simulink model "LPL_Hopper_Model"  (R2024b)
settings: Solver=VariableStepAuto  StartTime=0.0  StopTime=10.0  RelTol=1e-3
values from neighbouring files (symbols this model uses):
  S_Eb = [(-3/4)*He*me; 0; 0]    [HopperSimDriverScript.m]
  S_TD = [x_cg*mf; 0 ; 0]    [HopperSimDriverScript.m]
  THETA_IC = [0 0 0]    [HopperSimDriverScript.m]
  v_b_0 = [1 0 0]'    [HopperSimDriverScript.m]
libraries: matrix_library x5, sharedtransform x2, aerolibutil x1, sharedutil x1
settings Model: Creator=enson  LastModifiedBy=enson
settings RTWCC: GPUComputeCapability=3.5

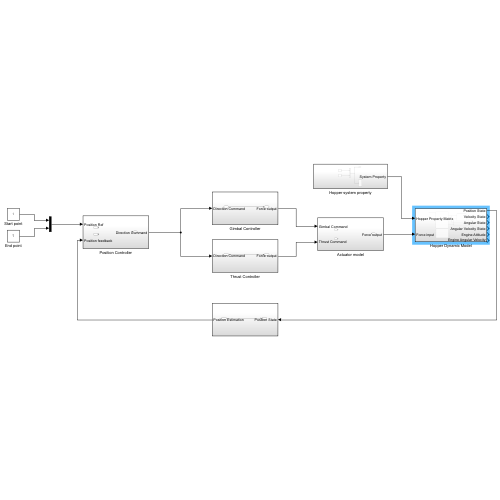
[thumbnail: Simulink's stored preview of the top-level diagram]
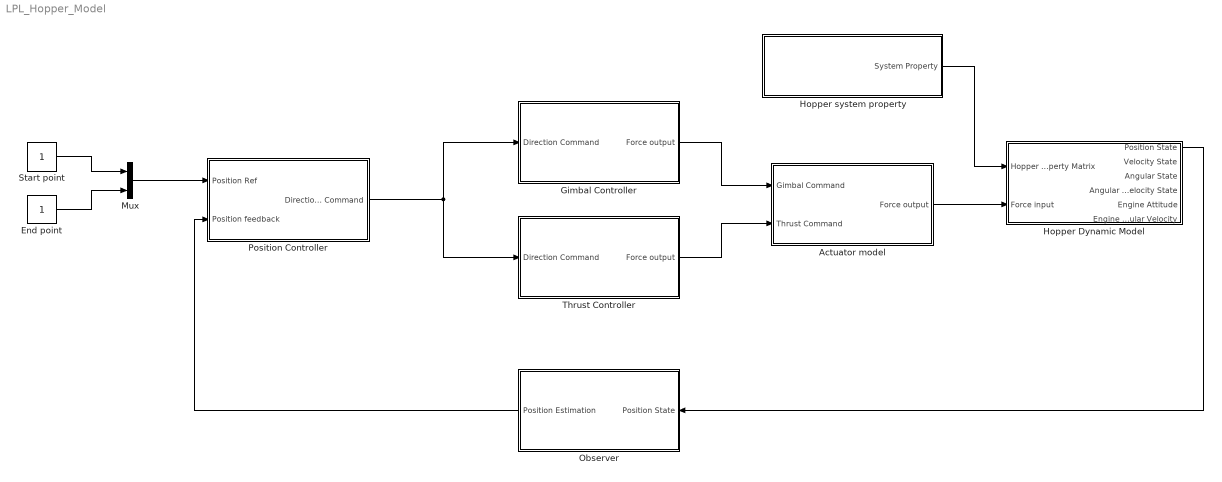
== system LPL_Hopper_Model ==
  Actuator model : Subsystem
  End point : Constant
  Gimbal Controller : Subsystem
  Hopper Dynamic Model : Subsystem
  Hopper system property : Subsystem
  Mux : Mux  Inputs=2
  Observer : Subsystem
  Position Controller : Subsystem
  Start point : Constant
  Thrust Controller : Subsystem
  wires:
  Mux/1 -> Position Controller/1(Position Ref)
  Start point/1 -> Mux/1
  End point/1 -> Mux/2
  Hopper Dynamic Model/1(Position State) -> Observer/1(Position State)
  Observer/1(Position Estimation) -> Position Controller/2(Position feedback)
  Position Controller/1(Direction Command) -> Gimbal Controller/1(Direction Command), Thrust Controller/1(Direction Command)
  Gimbal Controller/1(Force output) -> Actuator model/1(Gimbal Command)
  Thrust Controller/1(Force output) -> Actuator model/2(Thrust Command)
  Actuator model/1(Force output) -> Hopper Dynamic Model/2(Force input)
  Hopper system property/1(System Property) -> Hopper Dynamic Model/1(Hopper Property Matrix)

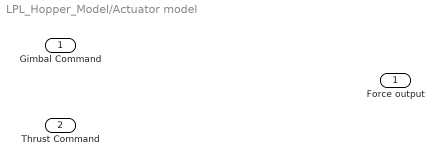
== system LPL_Hopper_Model/Actuator model ==
  Gimbal Command : Inport
  Thrust Command : Inport  Port=2
  Force output : Outport

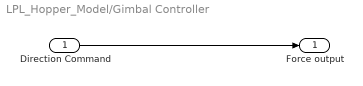
== system LPL_Hopper_Model/Gimbal Controller ==
  Direction Command : Inport
  Force output : Outport
  wires:
  Direction Command/1 -> Force output/1

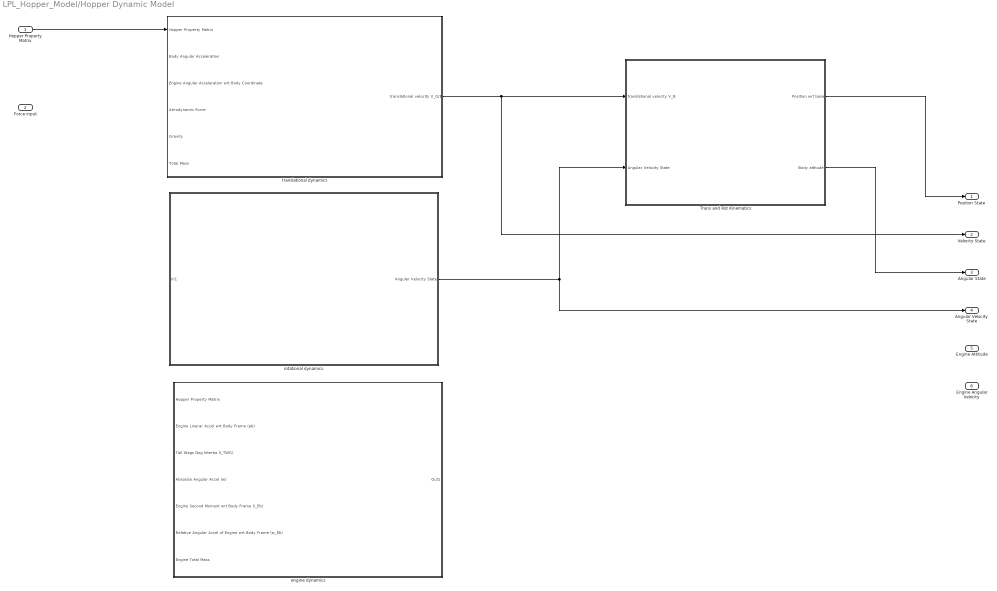
== system LPL_Hopper_Model/Hopper Dynamic Model ==
  Hopper Property Matrix : Inport
  Force input : Inport  Port=2
  Trans and Rot Kinematics : Subsystem
  engine dynamics : Subsystem
  rotational dynamics : Subsystem
  translational dynamics : Subsystem
  Position State : Outport
  Velocity State : Outport  Port=2
  Angular State : Outport  Port=3
  Angular Velocity State : Outport  Port=4
  Engine Attitude : Outport  Port=5
  Engine Angular Velocity : Outport  Port=6
  wires:
  Hopper Property Matrix/1 -> translational dynamics/1(Hopper Property Matrix)
  rotational dynamics/1(Angular Velocity State) -> Angular Velocity State/1, Trans and Rot Kinematics/2(Angular Velocity State)
  translational dynamics/1(translational velocity V_O/E) -> Velocity State/1, Trans and Rot Kinematics/1(translational velocity V_B)
  Trans and Rot Kinematics/1(Position wrt base) -> Position State/1
  Trans and Rot Kinematics/2(Body attitude) -> Angular State/1

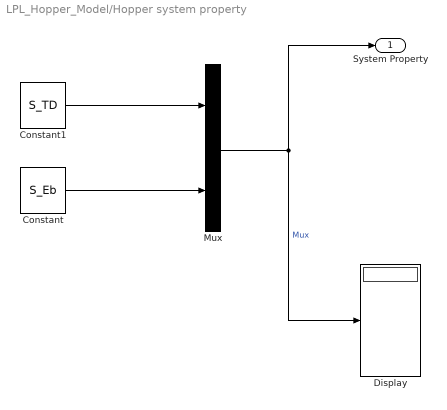
== system LPL_Hopper_Model/Hopper system property ==
  Constant : Constant  Value=S_Eb  VectorParams1D=off
  Constant1 : Constant  Value=S_TD  VectorParams1D=off
  Display : Display
  Mux : Mux  Inputs=2
  System Property : Outport
  wires:
  Mux/1 -> Display/1, System Property/1  "Mux"
  Constant/1 -> Mux/2
  Constant1/1 -> Mux/1

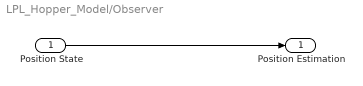
== system LPL_Hopper_Model/Observer ==
  Position State : Inport
  Position Estimation : Outport
  wires:
  Position State/1 -> Position Estimation/1

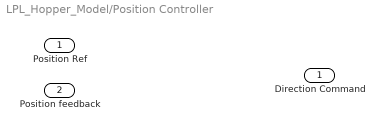
== system LPL_Hopper_Model/Position Controller ==
  Position Ref : Inport
  Position feedback : Inport  Port=2
  Direction Command : Outport

== system LPL_Hopper_Model/Thrust Controller ==
  Direction Command : Inport
  Force output : Outport
  wires:
  Direction Command/1 -> Force output/1

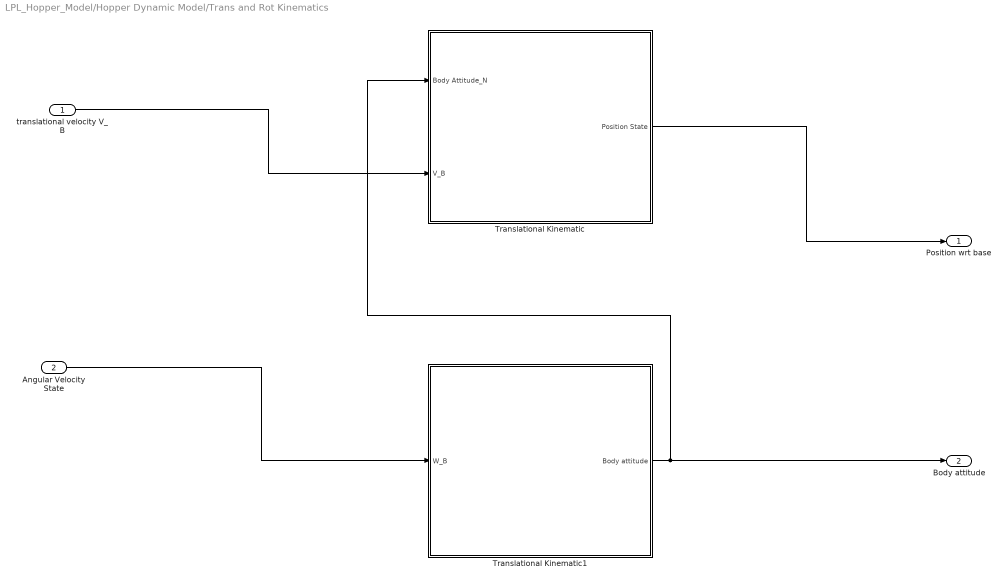
== system LPL_Hopper_Model/Hopper Dynamic Model/Trans and Rot Kinematics ==
  translational velocity V_B : Inport
  Angular Velocity State : Inport  Port=2
  Translational Kinematic : Subsystem
  Translational Kinematic1 : Subsystem
  Position wrt base : Outport
  Body attitude : Outport  Port=2
  wires:
  translational velocity V_B/1 -> Translational Kinematic/2(V_B)
  Translational Kinematic1/1(Body attitude) -> Body attitude/1, Translational Kinematic/1(Body Attitude_N)
  Angular Velocity State/1 -> Translational Kinematic1/1(W_B)
  Translational Kinematic/1(Position State) -> Position wrt base/1

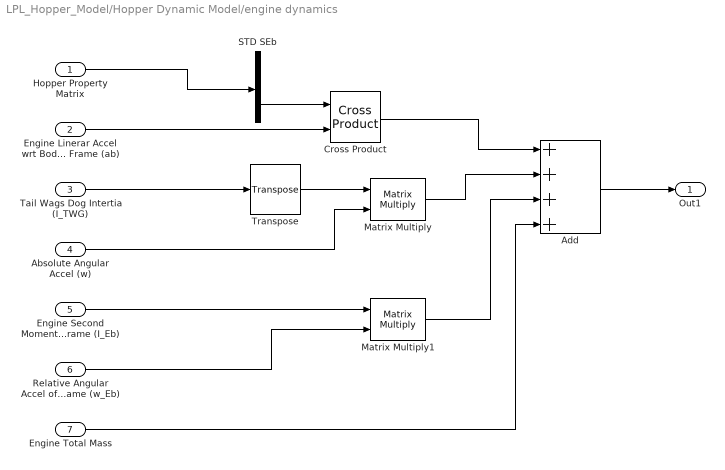
== system LPL_Hopper_Model/Hopper Dynamic Model/engine dynamics ==
  Hopper Property Matrix : Inport
  Engine Linerar Accel wrt Body Frame (ab) : Inport  Port=2
  Tail Wags Dog Intertia (I_TWG) : Inport  Port=3
  Absolute Angular Accel (w) : Inport  Port=4
  Engine Second Moment wrt Body Frame (I_Eb) : Inport  Port=5
  Relative Angular Accel of Engine wrt Body Frame (w_Eb) : Inport  Port=6
  Engine Total Mass : Inport  Port=7
  Add : Sum  Inputs=++++
  Cross Product : matrix_library/Cross Product
  Matrix Multiply : Product  Multiplication=Matrix(*)
  Matrix Multiply1 : Product  Multiplication=Matrix(*)
  STD SEb : Demux  Outputs=2
  Transpose : matrix_library/Transpose
  Out1 : Outport
  wires:
  Hopper Property Matrix/1 -> STD SEb/1
  STD SEb/2 -> Cross Product/1
  Engine Linerar Accel wrt Body Frame (ab)/1 -> Cross Product/2
  Cross Product/1 -> Add/1
  Tail Wags Dog Intertia (I_TWG)/1 -> Transpose/1
  Add/1 -> Out1/1
  Transpose/1 -> Matrix Multiply/1
  Absolute Angular Accel (w)/1 -> Matrix Multiply/2
  Matrix Multiply/1 -> Add/2
  Engine Second Moment wrt Body Frame (I_Eb)/1 -> Matrix Multiply1/1
  Relative Angular Accel of Engine wrt Body Frame (w_Eb)/1 -> Matrix Multiply1/2
  Matrix Multiply1/1 -> Add/3
  Engine Total Mass/1 -> Add/4

== system LPL_Hopper_Model/Hopper Dynamic Model/rotational dynamics ==
  In1 : Inport
  Angular Velocity State : Outport
  wires:
  In1/1 -> Angular Velocity State/1

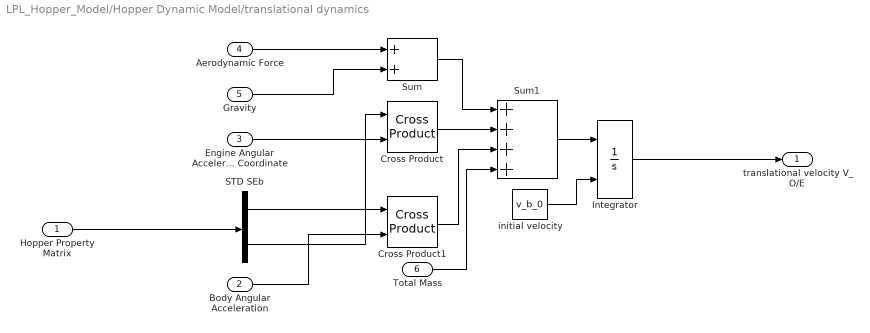
== system LPL_Hopper_Model/Hopper Dynamic Model/translational dynamics ==
  Hopper Property Matrix : Inport
  Body Angular Acceleration : Inport  Port=2
  Engine Angular Acceleration wrt Body Coordinate : Inport  Port=3
  Aerodynamic Force : Inport  Port=4
  Gravity : Inport  Port=5
  Total Mass : Inport  Port=6
  Cross Product : matrix_library/Cross Product
  Cross Product1 : matrix_library/Cross Product
  Integrator : Integrator  InitialConditionSource=external
  STD SEb : Demux  Outputs=2
  Sum : Sum
  Sum1 : Sum  Inputs=++++
  initial velocity : Constant  Value=v_b_0
  translational velocity V_O/E : Outport
  wires:
  Hopper Property Matrix/1 -> STD SEb/1
  Gravity/1 -> Sum/2
  Engine Angular Acceleration wrt Body Coordinate/1 -> Cross Product/2
  Aerodynamic Force/1 -> Sum/1
  STD SEb/2 -> Cross Product/1
  STD SEb/1 -> Cross Product1/1
  Body Angular Acceleration/1 -> Cross Product1/2
  Sum/1 -> Sum1/1
  Total Mass/1 -> Sum1/4
  Cross Product/1 -> Sum1/2
  Cross Product1/1 -> Sum1/3
  Sum1/1 -> Integrator/1
  initial velocity/1 -> Integrator/2
  Integrator/1 -> translational velocity V_O/E/1

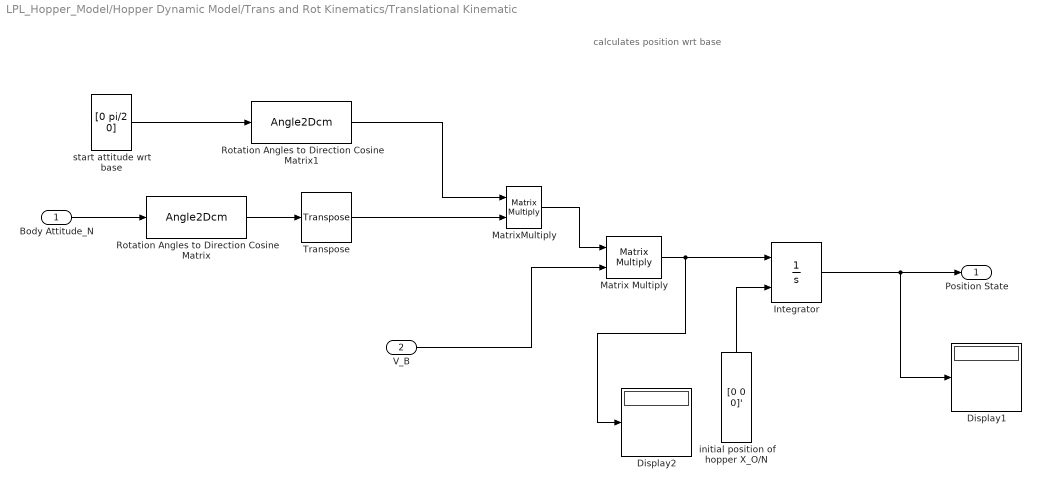
== system LPL_Hopper_Model/Hopper Dynamic Model/Trans and Rot Kinematics/Translational Kinematic ==
  note: calculates position wrt base
  Body Attitude_N : Inport
  V_B : Inport  Port=2
  Display1 : Display
  Display2 : Display
  Integrator : Integrator  InitialConditionSource=external
  Matrix Multiply : Product  Multiplication=Matrix(*)
  MatrixMultiply : Product  Multiplication=Matrix(*)
  Rotation Angles to Direction Cosine Matrix : Angle2Dcm
      settings: AttributesFormatString=Rotation Order: %<rotationOrder>
  Rotation Angles to Direction Cosine Matrix1 : Angle2Dcm
      settings: AttributesFormatString=Rotation Order: %<rotationOrder>
  Transpose : matrix_library/Transpose
  initial position of hopper X_O/N : Constant  Value=[0 0 0]'
  start attitude wrt base : Constant  Value=[0 pi/2 0]
  Position State : Outport
  wires:
  Matrix Multiply/1 -> Display2/1, Integrator/1
  initial position of hopper X_O/N/1 -> Integrator/2
  Integrator/1 -> Display1/1, Position State/1
  V_B/1 -> Matrix Multiply/2
  Body Attitude_N/1 -> Rotation Angles to Direction Cosine Matrix/1
  Rotation Angles to Direction Cosine Matrix/1 -> Transpose/1
  start attitude wrt base/1 -> Rotation Angles to Direction Cosine Matrix1/1
  Rotation Angles to Direction Cosine Matrix1/1 -> MatrixMultiply/1
  Transpose/1 -> MatrixMultiply/2
  MatrixMultiply/1 -> Matrix Multiply/1

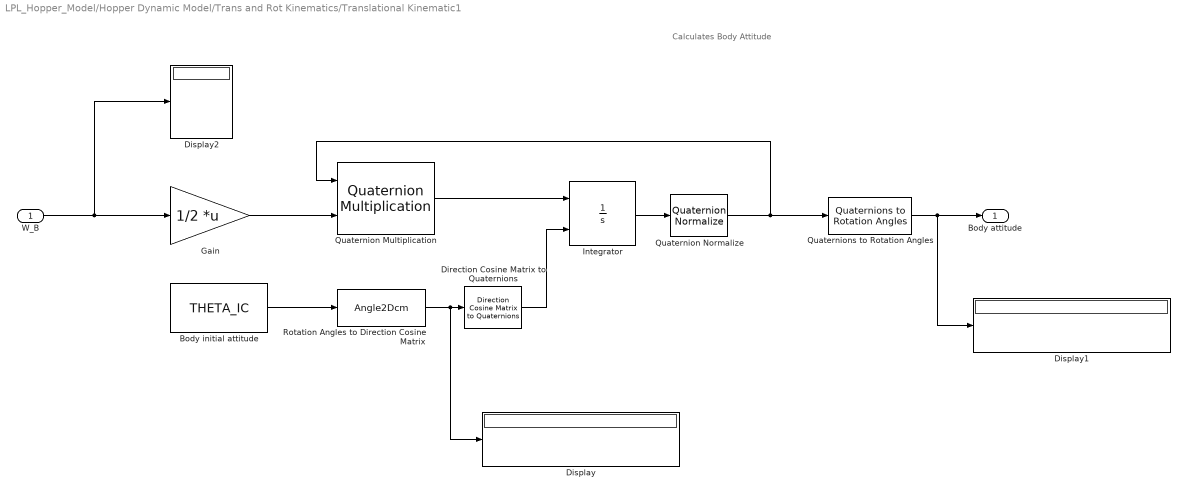
== system LPL_Hopper_Model/Hopper Dynamic Model/Trans and Rot Kinematics/Translational Kinematic1 ==
  note: Calculates Body Attitude
  W_B : Inport
  Body initial attitude : Constant  Value=THETA_IC  VectorParams1D=off
  Direction Cosine Matrix to Quaternions : sharedtransform/Direction Cosine Matrix  to Quaternions  aMode=0  action=None  tolerance=eps(2)
  Display : Display
  Display1 : Display
  Display2 : Display
  Gain : Gain  Gain=1/2  Multiplication=Matrix(K*u)
  Integrator : Integrator  InitialConditionSource=external
  Quaternion Multiplication : aerolibutil/Quaternion Multiplication
  Quaternion Normalize : sharedutil/Quaternion Normalize  aMode=aMode
  Quaternions to Rotation Angles : sharedtransform/Quaternions to Rotation Angles  rotationOrder=ZYX  aMode=aMode
  Rotation Angles to Direction Cosine Matrix : Angle2Dcm
      settings: AttributesFormatString=Rotation Order: %<rotationOrder>
  Body attitude : Outport
  wires:
  W_B/1 -> Display2/1, Gain/1
  Gain/1 -> Quaternion Multiplication/2
  Quaternion Multiplication/1 -> Integrator/1
  Integrator/1 -> Quaternion Normalize/1
  Quaternion Normalize/1 -> Quaternions to Rotation Angles/1, Quaternion Multiplication/1
  Quaternions to Rotation Angles/1 -> Display1/1, Body attitude/1
  Body initial attitude/1 -> Rotation Angles to Direction Cosine Matrix/1
  Rotation Angles to Direction Cosine Matrix/1 -> Display/1, Direction Cosine Matrix to Quaternions/1
  Direction Cosine Matrix to Quaternions/1 -> Integrator/2
